simulink model "observer_feedback"  (R2019a)
settings: Solver=VariableStepAuto  StartTime=0.0  StopTime=2  RelTol=1e-3
settings Model: Creator=harkib  LastModifiedBy=harki
settings DataIOCC: ReturnWorkspaceOutputs=off
settings DebuggingCC: ArithmeticOperatorsInVariantConditions=warning
settings SFSimCC: SimUseLocalCustomCode=off
settings RTWCC: RTWUseLocalCustomCode=off

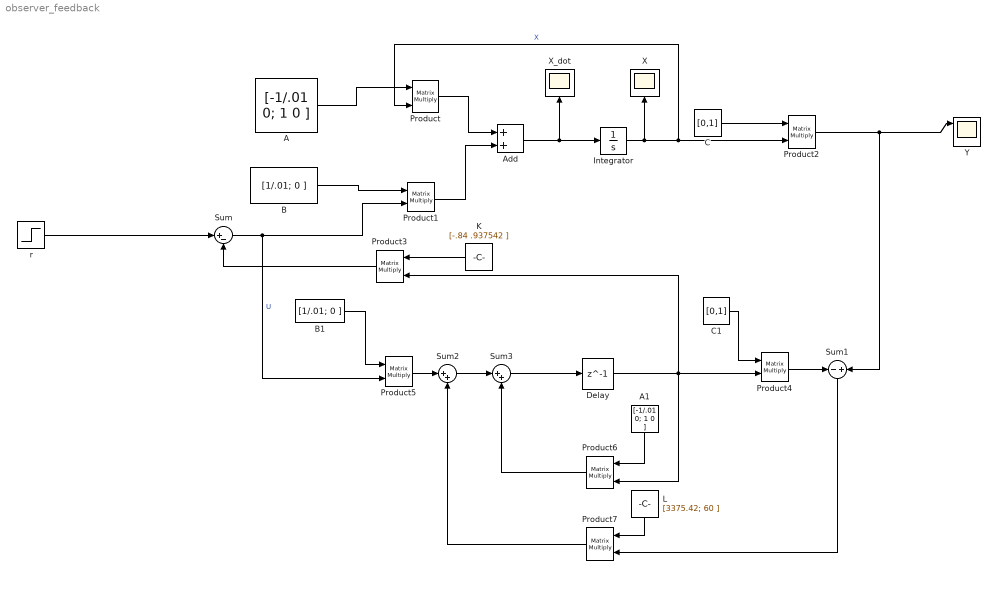
== system observer_feedback ==
  A : Constant  Value=[-1/.01 0; 1 0 ]  VectorParams1D=off
  A1 : Constant  Value=[-1/.01 0; 1 0 ]  VectorParams1D=off
  Add : Sum
  B : Constant  Value=[1/.01; 0 ]  VectorParams1D=off
  B1 : Constant  Value=[1/.01; 0 ]  VectorParams1D=off
  C : Constant  Value=[0,1]  VectorParams1D=off
  C1 : Constant  Value=[0,1]  VectorParams1D=off
  Delay : Delay  DelayLength=1  InitialCondition=0
  Integrator : Integrator
  K : Constant  Value=[-.84 .937542 ]  VectorParams1D=off
  L : Constant  Value=[3375.42; 60 ]  VectorParams1D=off
  Product{,1..7} (8 alike) : Product  Multiplication=Matrix(*)
  Sum : Sum  Inputs=|+-
  Sum1 : Sum  Inputs=-|+
  Sum2 : Sum  Inputs=|++
  Sum3 : Sum  Inputs=|++
  X : Scope
  X_dot : Scope
  Y : Scope  NumInputPorts=3
  r : Step  SampleTime=0
  wires:
  Add/1 -> X_dot/1, Integrator/1
  Product1/1 -> Add/2
  Product/1 -> Add/1
  B/1 -> Product1/1
  A/1 -> Product/1
  r/1 -> Sum/1
  K/1 -> Product3/1
  Integrator/1 -> Product2/2, Product/2, X/1  "X"
  Product3/1 -> Sum/2
  Sum/1 -> Product5/2, Product1/2  "U"
  C/1 -> Product2/1
  Product2/1 -> Sum1/2, Y/1
  Product4/1 -> Sum1/1
  C1/1 -> Product4/1
  B1/1 -> Product5/1
  Product5/1 -> Sum2/1
  Sum2/1 -> Sum3/1
  Delay/1 -> Product6/2, Product3/2, Product4/2
  Sum3/1 -> Delay/1
  A1/1 -> Product6/1
  Product6/1 -> Sum3/2
  Sum1/1 -> Product7/2
  L/1 -> Product7/1
  Product7/1 -> Sum2/2
